simulink model "DCMotor_T3_B_Simulink"  (R2024b)
settings: Solver=VariableStepAuto  StartTime=0.0  StopTime=10.0  RelTol=1e-3
values from neighbouring files (symbols this model uses):
  B = 1    [T2_A_T3_B.m]    (also in T2_B_T3_C.m = 0.01)
  Cu = 1    [T2_A_T3_B.m]
  J = 1    [T2_A_T3_B.m]
  L = 1    [T2_A_T3_B.m]
  p = [0, 0, 0]    [T1_B_T3_A.m]    (also in T2_A_T3_B.m = [0, 0]; T2_B_T3_C.m = [0, 1])
  R = 1    [T2_A_T3_B.m]
settings Model: Creator=lukiq  LastModifiedBy=lukiq

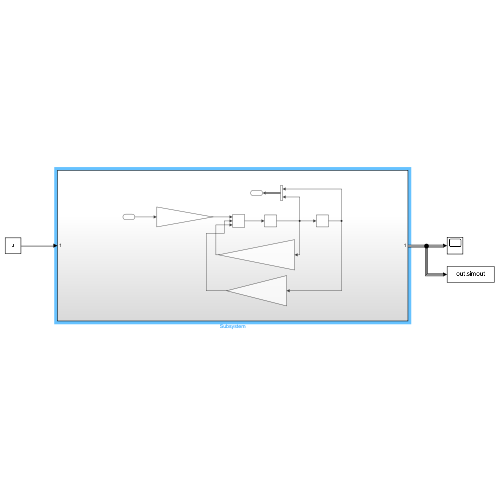
[thumbnail: Simulink's stored preview of the top-level diagram]
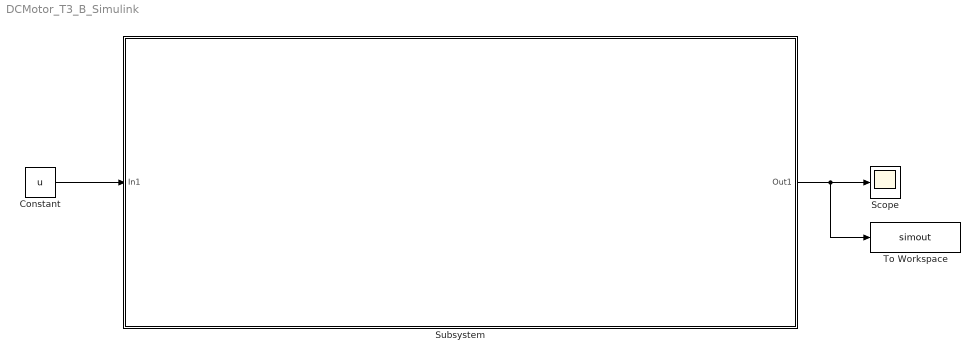
== system DCMotor_T3_B_Simulink ==
  Constant : Constant  Value=u
  Scope : Scope
  Subsystem : Subsystem
  To Workspace : ToWorkspace  VariableName=simout  SaveFormat=Timeseries  SampleTime=-1
  wires:
  Constant/1 -> Subsystem/1(In1)
  Subsystem/1(Out1) -> To Workspace/1, Scope/1

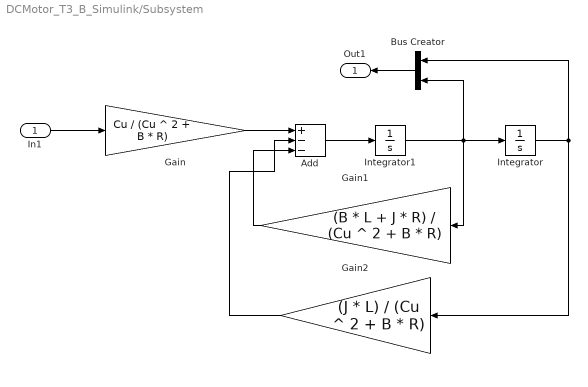
== system DCMotor_T3_B_Simulink/Subsystem ==
  In1 : Inport
  Add : Sum  Inputs=+--
  Bus Creator : BusCreator  Inputs=2
  Gain : Gain  Gain=Cu / (Cu ^ 2 + B * R)
  Gain1 : Gain  Gain=(B * L + J * R) / (Cu ^ 2 + B * R)
  Gain2 : Gain  Gain=(J * L) / (Cu ^ 2 + B * R)
  Integrator : Integrator  InitialCondition=p(1)
  Integrator1 : Integrator  InitialCondition=p(2)
  Out1 : Outport
  wires:
  Integrator1/1 -> Bus Creator/2, Integrator/1, Gain1/1
  Integrator/1 -> Bus Creator/1, Gain2/1
  In1/1 -> Gain/1
  Gain2/1 -> Add/2
  Gain1/1 -> Add/3
  Gain/1 -> Add/1
  Bus Creator/1 -> Out1/1
  Add/1 -> Integrator1/1
